simulink model "chap11_5sim"  (Simulink 10.3)
settings: Solver=ode45  StartTime=0.0  StopTime=10  FixedStep=0.00000010  RelTol=1e-3  EnableMultiTasking=on
settings Model: Creator=ljk  LastModifiedBy=shipe  ExtModeTrigMode=oneshot  ExtModeArmWhenConnect=off
settings OptimizationCC: BlockReduction=off  BooleanDataType=off
settings DebuggingCC: SaveWithParameterizedLinksMsg=none  SignalResolutionControl=TryResolveAllWithWarning  MultiTaskDSMMsg=warning  MultiTaskCondExecSysMsg=none
settings HardwareCC: TargetUnknown=on

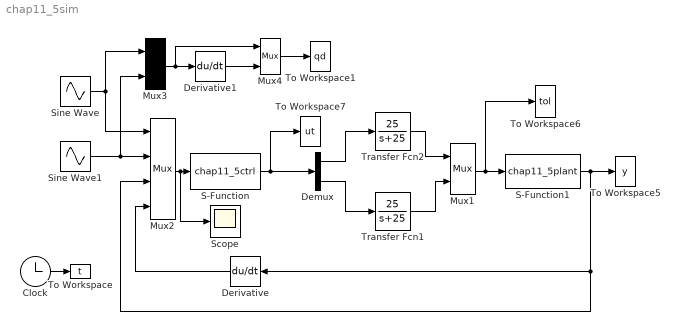
== system chap11_5sim ==
  Clock : Clock
  Demux : Demux  Outputs=2
  Derivative : Derivative
  Derivative1 : Derivative
  Mux1 : Mux  Inputs=2
  Mux2 : Mux
  Mux3 : Mux  Inputs=2
  Mux4 : Mux  Inputs=2
  S-Function : S-Function  FunctionName=chap11_5ctrl  SFunctionDeploymentMode=off  EnableBusSupport=off
  S-Function1 : S-Function  FunctionName=chap11_5plant  SFunctionDeploymentMode=off  EnableBusSupport=off
  Scope : Scope
  Sine Wave : Sin  Frequency=pi  SampleTime=0
  Sine Wave1 : Sin  Frequency=pi  Phase=pi/2  SampleTime=0
  To Workspace : ToWorkspace  VariableName=t  SampleTime=-1
  To Workspace1 : ToWorkspace  VariableName=qd  SampleTime=-1
  To Workspace5 : ToWorkspace  VariableName=y  SampleTime=-1
  To Workspace6 : ToWorkspace  VariableName=tol  SampleTime=-1
  To Workspace7 : ToWorkspace  VariableName=ut  SampleTime=-1
  Transfer Fcn1 : TransferFcn  Numerator=[25]  Denominator=[1 25]
  Transfer Fcn2 : TransferFcn  Numerator=[25]  Denominator=[1 25]
  wires:
  S-Function1/1 -> To Workspace5/1, Derivative/1, Mux2/3
  S-Function/1 -> To Workspace7/1, Demux/1
  Derivative/1 -> Mux2/4
  Sine Wave/1 -> Mux2/1, Mux3/1
  Sine Wave1/1 -> Mux2/2, Mux3/2
  Clock/1 -> To Workspace/1
  Mux2/1 -> Scope/1, S-Function/1
  Mux1/1 -> S-Function1/1, To Workspace6/1
  Transfer Fcn2/1 -> Mux1/1
  Transfer Fcn1/1 -> Mux1/2
  Demux/1 -> Transfer Fcn2/1
  Demux/2 -> Transfer Fcn1/1
  Derivative1/1 -> Mux4/2
  Mux3/1 -> Derivative1/1, Mux4/1
  Mux4/1 -> To Workspace1/1
